simulink model "EKFestes"  (R2017a)
settings: Solver=FixedStepDiscrete  StartTime=0.0  StopTime=3  FixedStep=0.001  RelTol=1e-3
libraries: dspsrcs4 x8
settings Model: Creator=Danie  LastModifiedBy=Danie

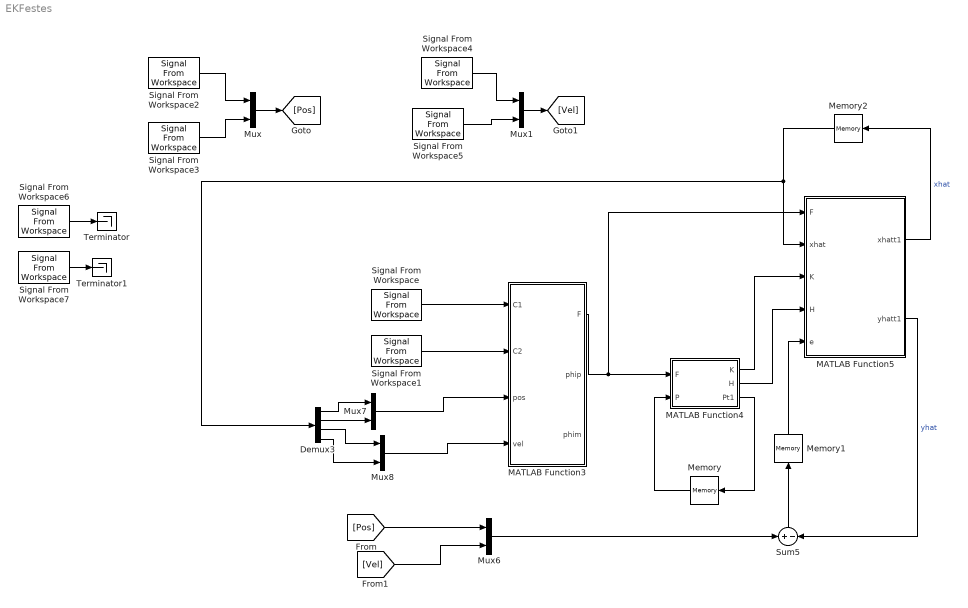
== system EKFestes ==
  Demux3 : Demux
  MATLAB Function3 : MATLAB Function  TreatAsAtomicUnit=on
  MATLAB Function4 : MATLAB Function  TreatAsAtomicUnit=on
  MATLAB Function5 : MATLAB Function  TreatAsAtomicUnit=on
  Memory : Memory  X0=eye(4)
  Memory1 : Memory  X0=zeros(4,1)
  Memory2 : Memory  X0=[1.75; 1.39; 0;0]
  Mux{,1,6..8} (5 alike) : Mux  Inputs=2
  Signal From Workspace : dspsrcs4/Signal From Workspace  X=C1  Ts=0.001  nsamps=1  OutputAfterFinalValue=Setting to zero  ignoreOrWarnInputAndFrameLengths=off  OutputFrames=off
  Signal From Workspace1 : dspsrcs4/Signal From Workspace  X=C2  Ts=0.001  nsamps=1  OutputAfterFinalValue=Setting to zero  ignoreOrWarnInputAndFrameLengths=off  OutputFrames=off
  Signal From Workspace2 : dspsrcs4/Signal From Workspace  X=pB  Ts=0.001  nsamps=1  OutputAfterFinalValue=Setting to zero  ignoreOrWarnInputAndFrameLengths=off  OutputFrames=off
  Signal From Workspace3 : dspsrcs4/Signal From Workspace  X=pA  Ts=0.001  nsamps=1  OutputAfterFinalValue=Setting to zero  ignoreOrWarnInputAndFrameLengths=off  OutputFrames=off
  Signal From Workspace4 : dspsrcs4/Signal From Workspace  X=Vb  Ts=0.001  nsamps=1  OutputAfterFinalValue=Setting to zero  ignoreOrWarnInputAndFrameLengths=off  OutputFrames=off
  Signal From Workspace5 : dspsrcs4/Signal From Workspace  X=Va  Ts=0.001  nsamps=1  OutputAfterFinalValue=Setting to zero  ignoreOrWarnInputAndFrameLengths=off  OutputFrames=off
  Signal From Workspace6 : dspsrcs4/Signal From Workspace  X=C1M  Ts=0.001  nsamps=1  OutputAfterFinalValue=Setting to zero  ignoreOrWarnInputAndFrameLengths=off  OutputFrames=off
  Signal From Workspace7 : dspsrcs4/Signal From Workspace  X=C2M  Ts=0.001  nsamps=1  OutputAfterFinalValue=Setting to zero  ignoreOrWarnInputAndFrameLengths=off  OutputFrames=off
  Sum5 : Sum  Inputs=+|-
  Terminator : Terminator
  Terminator1 : Terminator
  wires:
  Demux3/2 -> Mux7/2
  Mux8/1 -> MATLAB Function3/4(vel)
  MATLAB Function5/2(yhatt1) -> Sum5/2  "yhat"
  Memory1/1 -> MATLAB Function5/5(e)
  MATLAB Function5/1(xhatt1) -> Memory2/1  "xhat"
  MATLAB Function4/2(H) -> MATLAB Function5/4(H)
  MATLAB Function3/1(F) -> MATLAB Function5/1(F), MATLAB Function4/1(F)
  Memory2/1 -> Demux3/1, MATLAB Function5/2(xhat)
  Demux3/1 -> Mux7/1
  MATLAB Function4/1(K) -> MATLAB Function5/3(K)
  Sum5/1 -> Memory1/1
  Memory/1 -> MATLAB Function4/2(P)
  MATLAB Function4/3(Pt1) -> Memory/1
  Demux3/3 -> Mux8/1
  Mux6/1 -> Sum5/1
  Mux7/1 -> MATLAB Function3/3(pos)
  Demux3/4 -> Mux8/2
  Signal From Workspace/1 -> MATLAB Function3/1(C1)
  Signal From Workspace1/1 -> MATLAB Function3/2(C2)
  Signal From Workspace2/1 -> Mux/1
  Signal From Workspace3/1 -> Mux/2
  Signal From Workspace4/1 -> Mux1/1
  Signal From Workspace5/1 -> Mux1/2
  Mux/1 -> [Pos]
  Mux1/1 -> [Vel]
  [Pos] -> Mux6/1
  [Vel] -> Mux6/2
  Signal From Workspace6/1 -> Terminator/1
  Signal From Workspace7/1 -> Terminator1/1

== matlab function EKFestes/MATLAB Function3 ==
  data: C1 input; F output; C2 input; pos input; vel input; phip output; phim output
function [F,phip,phim] = fcn(C1,C2,pos,vel)

% velocità [asse B, asse A]

dt = 0.001;
deltaXi = 1e-5;
F = zeros(4);
Ident = eye(4);

%% Calcolo phi e F

    
    for i = 1:4
      fp = [pos;vel]+deltaXi*Ident(:,i);
      fm = [pos;vel]-deltaXi*Ident(:,i);
      
      [Mp,Kp] = DinamicaKalman(fp);
      [Mm,Km] = DinamicaKalman(fm);
      
      
phip = [zeros(2), eye(2); zeros(2), -Mp^-1*Kp]*fp + [zeros(2); Mp^-1]*[C1;C2];
phim = [zeros(2), eye(2); zeros(2), -Mm^-1*Km]*fm + [zeros(2); Mm^-1]*[C1;C2];

Fp = fp + phip*dt;
Fm = fm + phim*dt;

F(:,i) = (Fp-Fm)/(2*deltaXi);
    end

end

== matlab function EKFestes/MATLAB Function4 ==
  data: F input; K output; H output; P input; Pt1 output
function [K,H,Pt1] = fcn(F,P)
v1 = 1e-5;
v2 = 1e-5;
H = eye(4);

K = F*P*H'*(H*P*H'+v2)^-1;

Pt1 = F*P*F'-K*(H*P*H'+v2)*K'+v1;

end

== matlab function EKFestes/MATLAB Function5 ==
  data: F input; xhat input; K input; xhatt1 output; H input; yhatt1 output; e input
function [xhatt1, yhatt1] = fcn(F,xhat,K,H,e)

xhatt1 = F*xhat+K*e;

yhatt1 = H*xhatt1;

end
